simulink library "DEM_lib"  (Simulink 7.4)
settings: Solver=FixedStepDiscrete  StartTime=0.0  StopTime=Inf  FixedStep=0.001  RelTol=1e-3
undefined symbols (not defined in the file or in its folder): BCU_Drive_St, BCU_FastCharge_St, BCU_SlowCharge_St, COR_Fault_Bus, CTC_DefaultOffline_CtrCmd, CTC_DriveEmgyDcnct_CtrCmd, CTC_DriveOffline_CtrCmd, CTC_DriveOnline_CtrCmd, EHP_Fault_Bus, FCM_Fault_Bus, SCM_Fault_Bus
libraries: Defined_Functionality x82, simulink x2
(part 2 of 4)

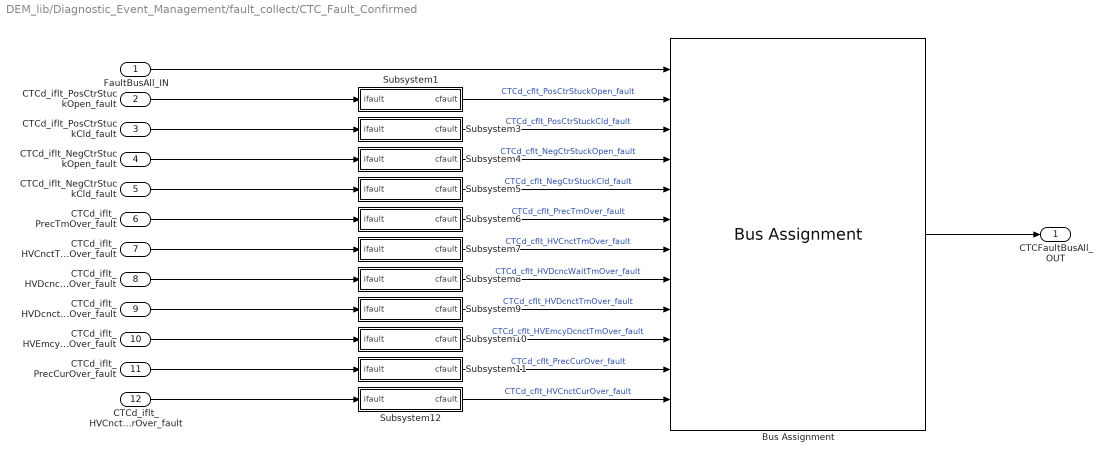
== system DEM_lib/Diagnostic_Event_Management/fault_collect/CTC_Fault_Confirmed ==
  FaultBusAll_IN : Inport
  CTCd_iflt_PosCtrStuckOpen_fault : Inport  Port=2
  CTCd_iflt_PosCtrStuckCld_fault : Inport  Port=3
  CTCd_iflt_NegCtrStuckOpen_fault : Inport  Port=4
  CTCd_iflt_NegCtrStuckCld_fault : Inport  Port=5
  CTCd_iflt_PrecTmOver_fault : Inport  Port=6
  CTCd_iflt_HVCnctTmOver_fault : Inport  Port=7
  CTCd_iflt_HVDcncWaitTmOver_fault : Inport  Port=8
  CTCd_iflt_HVDcnctTmOver_fault : Inport  Port=9
  CTCd_iflt_HVEmcyDcnctTmOver_fault : Inport  Port=10
  CTCd_iflt_PrecCurOver_fault : Inport  Port=11
  CTCd_iflt_HVCnctCurOver_fault : Inport  Port=12
  Bus Assignment : BusAssignment  Description=|  AssignedSignals=CTC_Fault_Bus.CTCd_cflt_PosCtrStuckOpen_faultRaw,CTC_Fault_Bus.CTCd_cflt_PosCtrStuckCld_faultRaw,CTC_Fault_Bus.CTCd_cflt_NegCtrStuckOpen_faultRaw,CTC_Fault_Bus.CTCd_cflt_NegCtrStuckCld_faultRaw,CTC_Fault_Bus.CTCd_cflt_PrecTmOver_faultRaw,CTC_Fault_Bus.CTCd_cflt_HVCnctTmOver_faultRaw,CTC_Fault_Bus.CTCd_cflt_HVDcncWaitTmOver_faultRaw,CTC_Fault_Bus.CTCd_cflt_HVDcnctTmOver_faultRaw,CTC_Fault_Bus.CTCd_cflt_HVEmcyDcnctTmOver_faultRaw,CTC_Fault_Bus.CTCd_cflt_PrecCurOver_faultRaw,CTC_Fault_Bus.CTCd_cflt_HVCnctCurOver_faultRaw
      | $Author:Yan LiJuan$
      | $Date:2015/03/26$  
      | $Revision:1.0$
  Subsystem1 : Subsystem
  Subsystem10 : Subsystem
  Subsystem11 : Subsystem
  Subsystem12 : Subsystem
  Subsystem3 : Subsystem
  Subsystem4 : Subsystem
  Subsystem5 : Subsystem
  Subsystem6 : Subsystem
  Subsystem7 : Subsystem
  Subsystem8 : Subsystem
  Subsystem9 : Subsystem
  CTCFaultBusAll_OUT : Outport
  wires:
  Subsystem12/1(cfault) -> Bus Assignment/12  "CTCd_cflt_HVCnctCurOver_fault"
  Subsystem11/1(cfault) -> Bus Assignment/11  "CTCd_cflt_PrecCurOver_fault"
  Subsystem10/1(cfault) -> Bus Assignment/10  "CTCd_cflt_HVEmcyDcnctTmOver_fault"
  Subsystem9/1(cfault) -> Bus Assignment/9  "CTCd_cflt_HVDcnctTmOver_fault"
  Subsystem8/1(cfault) -> Bus Assignment/8  "CTCd_cflt_HVDcncWaitTmOver_fault"
  Subsystem7/1(cfault) -> Bus Assignment/7  "CTCd_cflt_HVCnctTmOver_fault"
  Subsystem6/1(cfault) -> Bus Assignment/6  "CTCd_cflt_PrecTmOver_fault"
  Subsystem5/1(cfault) -> Bus Assignment/5  "CTCd_cflt_NegCtrStuckCld_fault"
  Subsystem4/1(cfault) -> Bus Assignment/4  "CTCd_cflt_NegCtrStuckOpen_fault"
  Subsystem3/1(cfault) -> Bus Assignment/3  "CTCd_cflt_PosCtrStuckCld_fault"
  Subsystem1/1(cfault) -> Bus Assignment/2  "CTCd_cflt_PosCtrStuckOpen_fault"
  Bus Assignment/1 -> CTCFaultBusAll_OUT/1
  CTCd_iflt_HVCnctCurOver_fault/1 -> Subsystem12/1(ifault)
  CTCd_iflt_PrecCurOver_fault/1 -> Subsystem11/1(ifault)
  CTCd_iflt_HVEmcyDcnctTmOver_fault/1 -> Subsystem10/1(ifault)
  CTCd_iflt_HVDcnctTmOver_fault/1 -> Subsystem9/1(ifault)
  CTCd_iflt_HVDcncWaitTmOver_fault/1 -> Subsystem8/1(ifault)
  CTCd_iflt_HVCnctTmOver_fault/1 -> Subsystem7/1(ifault)
  CTCd_iflt_PrecTmOver_fault/1 -> Subsystem6/1(ifault)
  CTCd_iflt_NegCtrStuckCld_fault/1 -> Subsystem5/1(ifault)
  CTCd_iflt_NegCtrStuckOpen_fault/1 -> Subsystem4/1(ifault)
  CTCd_iflt_PosCtrStuckCld_fault/1 -> Subsystem3/1(ifault)
  CTCd_iflt_PosCtrStuckOpen_fault/1 -> Subsystem1/1(ifault)
  FaultBusAll_IN/1 -> Bus Assignment/1

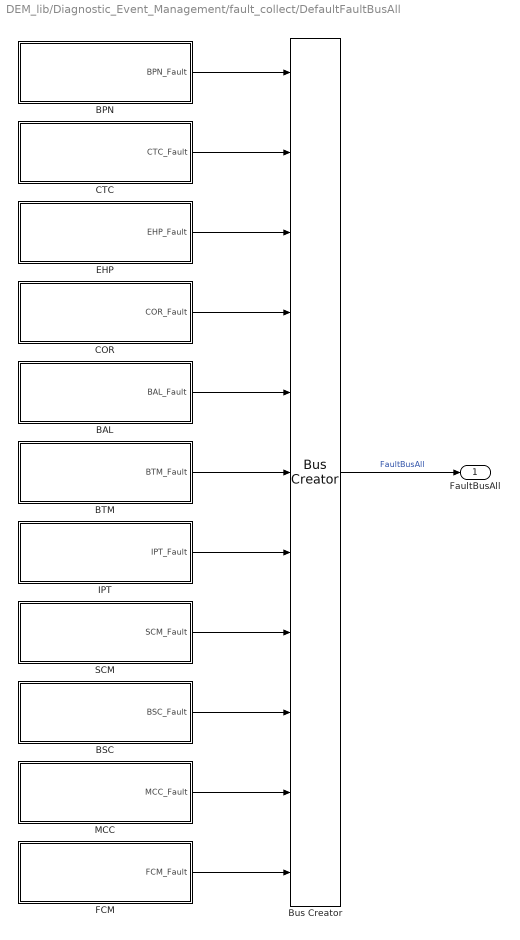
== system DEM_lib/Diagnostic_Event_Management/fault_collect/DefaultFaultBusAll ==
  BAL : Subsystem  Description=|
      | $Author:Yan LiJuan$
      | $Date:2015/03/26$  
      | $Revision:1.0$
  BPN : Subsystem  Description=|
      | $Author:Yan LiJuan$
      | $Date:2015/03/26$  
      | $Revision:1.0$
  BSC : Subsystem  Description=|
      | $Author:Yan LiJuan$
      | $Date:2015/03/26$  
      | $Revision:1.0$
  BTM : Subsystem  Description=|
      | $Author:Yan LiJuan$
      | $Date:2015/03/26$  
      | $Revision:1.0$
  Bus Creator : BusCreator  Inputs=11
  COR : Subsystem  Description=|
      | $Author:Yan LiJuan$
      | $Date:2015/03/26$  
      | $Revision:1.0$
  CTC : Subsystem  Description=|
      | $Author:Yan LiJuan$
      | $Date:2015/03/26$  
      | $Revision:1.0$
  EHP : Subsystem  Description=|
      | $Author:Yan LiJuan$
      | $Date:2015/03/26$  
      | $Revision:1.0$
  FCM : Subsystem  Description=|
      | $Author:Yan LiJuan$
      | $Date:2015/03/26$  
      | $Revision:1.0$
  IPT : Subsystem  Description=|
      | $Author:Yan LiJuan$
      | $Date:2015/03/26$  
      | $Revision:1.0$
  MCC : Subsystem  Description=|
      | $Author:Yan LiJuan$
      | $Date:2015/03/26$  
      | $Revision:1.0$
  SCM : Subsystem  Description=|
      | $Author:Yan LiJuan$
      | $Date:2015/03/26$  
      | $Revision:1.0$
  FaultBusAll : Outport  OutDataType=fixdt(1, 16)  OutScaling=2^0
  wires:
  FCM/1(FCM_Fault) -> Bus Creator/11
  BSC/1(BSC_Fault) -> Bus Creator/9
  SCM/1(SCM_Fault) -> Bus Creator/8
  Bus Creator/1 -> FaultBusAll/1  "FaultBusAll"
  IPT/1(IPT_Fault) -> Bus Creator/7
  BTM/1(BTM_Fault) -> Bus Creator/6
  BAL/1(BAL_Fault) -> Bus Creator/5
  COR/1(COR_Fault) -> Bus Creator/4
  EHP/1(EHP_Fault) -> Bus Creator/3
  CTC/1(CTC_Fault) -> Bus Creator/2
  BPN/1(BPN_Fault) -> Bus Creator/1
  MCC/1(MCC_Fault) -> Bus Creator/10

== system DEM_lib/Diagnostic_Event_Management/fault_collect/EHP_Fault_Confirmed ==
  FaultBusAll_IN : Inport
  EHPd_iflt_NegIso_fault : Inport  Port=2
  EHPd_iflt_NegIso_warn : Inport  Port=3
  EHPd_iflt_PosIso_fault : Inport  Port=4
  EHPd_iflt_PosIso_warn : Inport  Port=5
  EHPd_iflt_HVILSt_fault : Inport  Port=6
  Bus Assignment : BusAssignment  Description=|  AssignedSignals=EHP_Fault_Bus.EHPd_cflt_NegIso_faultRaw,EHP_Fault_Bus.EHPd_cflt_NegIso_warnRaw,EHP_Fault_Bus.EHPd_cflt_PosIso_faultRaw,EHP_Fault_Bus.EHPd_cflt_PosIso_warnRaw,EHP_Fault_Bus.EHPd_cflt_HVILSt_faultRaw
      | $Author:Yan LiJuan$
      | $Date:2015/03/26$  
      | $Revision:1.0$
  Subsystem2 : Subsystem
  Subsystem4 : Subsystem
  Subsystem5 : Subsystem
  Subsystem6 : Subsystem
  Subsystem7 : Subsystem
  EHPFaultBusAll_OUT : Outport
  wires:
  Subsystem7/1(cfault) -> Bus Assignment/6  "EHPd_cflt_HVILSt_fault"
  Subsystem6/1(cfault) -> Bus Assignment/5  "EHPd_cflt_PosIso_warn"
  Subsystem5/1(cfault) -> Bus Assignment/4  "EHPd_cflt_PosIso_fault"
  Subsystem4/1(cfault) -> Bus Assignment/3  "EHPd_cflt_NegIso_warn"
  Subsystem2/1(cfault) -> Bus Assignment/2  "EHPd_cflt_NegIso_fault"
  EHPd_iflt_HVILSt_fault/1 -> Subsystem7/1(ifault)
  EHPd_iflt_PosIso_warn/1 -> Subsystem6/1(ifault)
  EHPd_iflt_PosIso_fault/1 -> Subsystem5/1(ifault)
  EHPd_iflt_NegIso_warn/1 -> Subsystem4/1(ifault)
  EHPd_iflt_NegIso_fault/1 -> Subsystem2/1(ifault)
  Bus Assignment/1 -> EHPFaultBusAll_OUT/1
  FaultBusAll_IN/1 -> Bus Assignment/1

== system DEM_lib/Diagnostic_Event_Management/fault_collect/FCM_Fault_Confirmed ==
  FaultBusAll_IN : Inport
  FCMd_iflt_ChaCurDifOver_fault : Inport  Port=2
  FCMd_iflt_ChaVoltDifOver_fault : Inport  Port=3
  Bus Assignment : BusAssignment  Description=|  AssignedSignals=FCM_Fault_Bus.FCMd_cflt_ChaCurDifOver_faultRaw,FCM_Fault_Bus.FCMd_cflt_ChaVoltDifOver_faultRaw
      | $Author:Yan LiJuan$
      | $Date:2015/03/26$  
      | $Revision:1.0$
  Subsystem1 : Subsystem
  Subsystem2 : Subsystem
  FCMIPTFaultBusAll_OUT : Outport
  wires:
  Subsystem2/1(cfault) -> Bus Assignment/2  "FCMd_cflt_ChaCurDifOver_fault"
  Subsystem1/1(cfault) -> Bus Assignment/3  "FCMd_cflt_ChaVoltDifOver_fault"
  FCMd_iflt_ChaVoltDifOver_fault/1 -> Subsystem1/1(ifault)
  FCMd_iflt_ChaCurDifOver_fault/1 -> Subsystem2/1(ifault)
  Bus Assignment/1 -> FCMIPTFaultBusAll_OUT/1  "FCMIPTFaultBusAll_OUT"
  FaultBusAll_IN/1 -> Bus Assignment/1

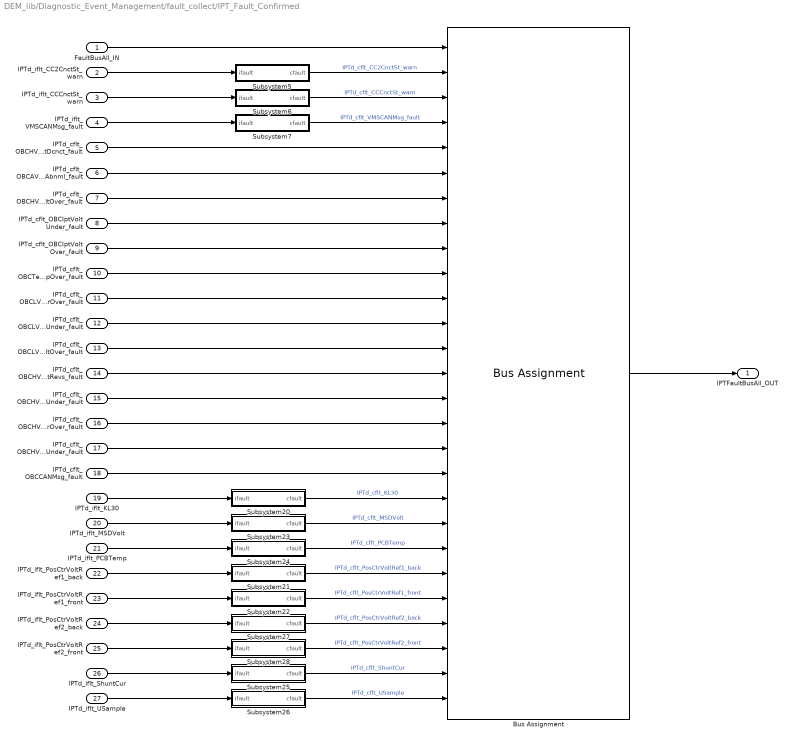
== system DEM_lib/Diagnostic_Event_Management/fault_collect/IPT_Fault_Confirmed ==
  FaultBusAll_IN : Inport
  IPTd_iflt_CC2CnctSt_warn : Inport  Port=2
  IPTd_iflt_CCCnctSt_warn : Inport  Port=3
  IPTd_iflt_VMSCANMsg_fault : Inport  Port=4
  IPTd_cflt_OBCHVOptDcnct_fault : Inport  Port=5  OutDataType=fixdt(1, 16)  OutScaling=2^0
  IPTd_cflt_OBCAVOptVoltAbnml_fault : Inport  Port=6  OutDataType=fixdt(1, 16)  OutScaling=2^0
  IPTd_cflt_OBCHVOptVoltOver_fault : Inport  Port=7  OutDataType=fixdt(1, 16)  OutScaling=2^0
  IPTd_cflt_OBCIptVoltUnder_fault : Inport  Port=8  OutDataType=fixdt(1, 16)  OutScaling=2^0
  IPTd_cflt_OBCIptVoltOver_fault : Inport  Port=9  OutDataType=fixdt(1, 16)  OutScaling=2^0
  IPTd_cflt_OBCTempOver_fault : Inport  Port=10  OutDataType=fixdt(1, 16)  OutScaling=2^0
  IPTd_cflt_OBCLVOptCurOver_fault : Inport  Port=11  OutDataType=fixdt(1, 16)  OutScaling=2^0
  IPTd_cflt_OBCLVOptVoltUnder_fault : Inport  Port=12  OutDataType=fixdt(1, 16)  OutScaling=2^0
  IPTd_cflt_OBCLVOptVoltOver_fault : Inport  Port=13  OutDataType=fixdt(1, 16)  OutScaling=2^0
  IPTd_cflt_OBCHVOptRevs_fault : Inport  Port=14  OutDataType=fixdt(1, 16)  OutScaling=2^0
  IPTd_cflt_OBCHVOptCurUnder_fault : Inport  Port=15  OutDataType=fixdt(1, 16)  OutScaling=2^0
  IPTd_cflt_OBCHVOptCurOver_fault : Inport  Port=16  OutDataType=fixdt(1, 16)  OutScaling=2^0
  IPTd_cflt_OBCHVOptVoltUnder_fault : Inport  Port=17  OutDataType=fixdt(1, 16)  OutScaling=2^0
  IPTd_cflt_OBCCANMsg_fault : Inport  Port=18  OutDataType=fixdt(1, 16)  OutScaling=2^0
  IPTd_iflt_KL30 : Inport  Port=19  OutDataType=fixdt(1, 16)  OutScaling=2^0
  IPTd_iflt_MSDVolt : Inport  Port=20  OutDataType=fixdt(1, 16)  OutScaling=2^0
  IPTd_iflt_PCBTemp : Inport  Port=21  OutDataType=fixdt(1, 16)  OutScaling=2^0
  IPTd_iflt_PosCtrVoltRef1_back : Inport  Port=22  OutDataType=fixdt(1, 16)  OutScaling=2^0
  IPTd_iflt_PosCtrVoltRef1_front : Inport  Port=23  OutDataType=fixdt(1, 16)  OutScaling=2^0
  IPTd_iflt_PosCtrVoltRef2_back : Inport  Port=24  OutDataType=fixdt(1, 16)  OutScaling=2^0
  IPTd_iflt_PosCtrVoltRef2_front : Inport  Port=25  OutDataType=fixdt(1, 16)  OutScaling=2^0
  IPTd_iflt_ShuntCur : Inport  Port=26  OutDataType=fixdt(1, 16)  OutScaling=2^0
  IPTd_iflt_USample : Inport  Port=27  OutDataType=fixdt(1, 16)  OutScaling=2^0
  Bus Assignment : BusAssignment  Description=|  AssignedSignals=IPT_Fault_Bus.IPTd_cflt_CC2CnctSt_warnRaw,IPT_Fault_Bus.IPTd_cflt_CCCnctSt_warnRaw,IPT_Fault_Bus.IPTd_cflt_VMSCANMsg_faultRaw,IPT_Fault_Bus.IPTd_cflt_OBCHVOptDcnct_faultRaw,IPT_Fault_Bus.IPTd_cflt_OBCAVOptVoltAbnml_faultRaw,IPT_Fault_Bus.IPTd_cflt_OBCHVOptVoltOver_faultRaw,IPT_Fault_Bus.IPTd_cflt_OBCIptVoltUnder_faultRaw,IPT_Fault_Bus.IPTd_cflt_OBCIptVoltOver_faultRaw,IPT_Fault_Bus.IPTd_cflt_OBCTempOver_faultRaw,IPT_Fault_Bus.IPTd_cflt_OBCLVOptCurOver_faultRaw,IPT_Fault_Bus.IPTd_cflt_OBCLVOptVoltUnder_faultRaw,IPT_Fault_Bus.IPTd_cflt_OBCLVOptVoltOver_faultRaw,IPT_Fault_Bus.IPTd_cflt_OBCHVOptRevs_faultRaw,IPT_Fault_Bus.IPTd_cflt_OBCHVOptCurUnder_faultRaw,IPT_Fault_Bus.IPTd_cflt_OBCHVOptCurOver_faultRaw,IPT_Fault_Bus.IPTd_cflt_OBCHVOptVoltUnder_faultRaw,IPT_Fault_Bus.IPTd_cflt_OBCCANMsg_faultRaw,IPT_Fault_Bus.IPTd_cflt_KL30Raw,IPT_Fault_Bus.IPTd_cflt_MSDVoltRaw,IPT_Fault_Bus.IPTd_cflt_PCBTempRaw,IPT_Fault_Bus.IPTd_cflt_PosCtrVoltRef1_backRaw,IPT_Fault_Bus.IPTd_cflt_PosCtrVoltRef1_frontRaw,IPT_Fault_Bus.IPTd_cflt_PosCtrVoltRef2_backRaw,IPT_Fault_Bus.IPTd_cflt_PosCtrVoltRef2_frontRaw,IPT_Fault_Bus.IPTd_cflt_ShuntCurRaw,IPT_Fault_Bus.IPTd_cflt_USampleRaw
      | $Author:Yan LiJuan$
      | $Date:2015/03/26$  
      | $Revision:1.0$
  Subsystem20 : Subsystem
  Subsystem21 : Subsystem
  Subsystem22 : Subsystem
  Subsystem23 : Subsystem
  Subsystem24 : Subsystem
  Subsystem25 : Subsystem
  Subsystem26 : Subsystem
  Subsystem27 : Subsystem
  Subsystem28 : Subsystem
  Subsystem5 : Subsystem
  Subsystem6 : Subsystem
  Subsystem7 : Subsystem
  IPTFaultBusAll_OUT : Outport
  wires:
  IPTd_cflt_OBCAVOptVoltAbnml_fault/1 -> Bus Assignment/6
  IPTd_cflt_OBCHVOptDcnct_fault/1 -> Bus Assignment/5
  Subsystem7/1(cfault) -> Bus Assignment/4  "IPTd_cflt_VMSCANMsg_fault"
  Subsystem6/1(cfault) -> Bus Assignment/3  "IPTd_cflt_CCCnctSt_warn"
  Subsystem5/1(cfault) -> Bus Assignment/2  "IPTd_cflt_CC2CnctSt_warn"
  IPTd_iflt_VMSCANMsg_fault/1 -> Subsystem7/1(ifault)
  IPTd_iflt_CCCnctSt_warn/1 -> Subsystem6/1(ifault)
  IPTd_iflt_CC2CnctSt_warn/1 -> Subsystem5/1(ifault)
  Bus Assignment/1 -> IPTFaultBusAll_OUT/1
  FaultBusAll_IN/1 -> Bus Assignment/1
  Subsystem20/1(cfault) -> Bus Assignment/19  "IPTd_cflt_KL30"
  Subsystem23/1(cfault) -> Bus Assignment/20  "IPTd_cflt_MSDVolt"
  Subsystem24/1(cfault) -> Bus Assignment/21  "IPTd_cflt_PCBTemp"
  Subsystem21/1(cfault) -> Bus Assignment/22  "IPTd_cflt_PosCtrVoltRef1_back"
  Subsystem22/1(cfault) -> Bus Assignment/23  "IPTd_cflt_PosCtrVoltRef1_front"
  Subsystem27/1(cfault) -> Bus Assignment/24  "IPTd_cflt_PosCtrVoltRef2_back"
  Subsystem28/1(cfault) -> Bus Assignment/25  "IPTd_cflt_PosCtrVoltRef2_front"
  Subsystem25/1(cfault) -> Bus Assignment/26  "IPTd_cflt_ShuntCur"
  Subsystem26/1(cfault) -> Bus Assignment/27  "IPTd_cflt_USample"
  IPTd_iflt_KL30/1 -> Subsystem20/1(ifault)
  IPTd_iflt_MSDVolt/1 -> Subsystem23/1(ifault)
  IPTd_iflt_PCBTemp/1 -> Subsystem24/1(ifault)
  IPTd_iflt_PosCtrVoltRef1_back/1 -> Subsystem21/1(ifault)
  IPTd_iflt_PosCtrVoltRef1_front/1 -> Subsystem22/1(ifault)
  IPTd_iflt_PosCtrVoltRef2_back/1 -> Subsystem27/1(ifault)
  IPTd_iflt_PosCtrVoltRef2_front/1 -> Subsystem28/1(ifault)
  IPTd_iflt_ShuntCur/1 -> Subsystem25/1(ifault)
  IPTd_iflt_USample/1 -> Subsystem26/1(ifault)
  IPTd_cflt_OBCHVOptVoltOver_fault/1 -> Bus Assignment/7
  IPTd_cflt_OBCIptVoltUnder_fault/1 -> Bus Assignment/8
  IPTd_cflt_OBCIptVoltOver_fault/1 -> Bus Assignment/9
  IPTd_cflt_OBCTempOver_fault/1 -> Bus Assignment/10
  IPTd_cflt_OBCLVOptCurOver_fault/1 -> Bus Assignment/11
  IPTd_cflt_OBCLVOptVoltUnder_fault/1 -> Bus Assignment/12
  IPTd_cflt_OBCLVOptVoltOver_fault/1 -> Bus Assignment/13
  IPTd_cflt_OBCHVOptRevs_fault/1 -> Bus Assignment/14
  IPTd_cflt_OBCHVOptCurUnder_fault/1 -> Bus Assignment/15
  IPTd_cflt_OBCHVOptCurOver_fault/1 -> Bus Assignment/16
  IPTd_cflt_OBCHVOptVoltUnder_fault/1 -> Bus Assignment/17
  IPTd_cflt_OBCCANMsg_fault/1 -> Bus Assignment/18

== system DEM_lib/Diagnostic_Event_Management/fault_collect/MCC_Fault_Confirmed ==
  FaultBusAll_IN : Inport
  MCCd_iflt_BMUInit_fault : Inport  Port=2
  Bus Assignment : BusAssignment  Description=|  AssignedSignals=MCC_Fault_Bus.MCCd_cflt_BMUInit_faultRaw
      | $Author:Yan LiJuan$
      | $Date:2015/03/26$  
      | $Revision:1.0$
  Subsystem2 : Subsystem
  MCCFaultBusAll_OUT : Outport
  wires:
  FaultBusAll_IN/1 -> Bus Assignment/1
  Bus Assignment/1 -> MCCFaultBusAll_OUT/1  "MCCFaultBusAll_OUT"
  MCCd_iflt_BMUInit_fault/1 -> Subsystem2/1(ifault)
  Subsystem2/1(cfault) -> Bus Assignment/2  "MCCd_cflt_BMUInit_fault"

== system DEM_lib/Diagnostic_Event_Management/fault_collect/SCM_Fault_Confirmed ==
  FaultBusAll_IN : Inport
  SCMd_iflt_CurOver_fault : Inport  Port=2
  SCMd_iflt_VoltOver_fault : Inport  Port=3
  Bus Assignment : BusAssignment  Description=|  AssignedSignals=SCM_Fault_Bus.SCMd_cflt_CurOver_faultRaw,SCM_Fault_Bus.SCMd_cflt_VoltOver_faultRaw
      | $Author:Yan LiJuan$
      | $Date:2015/03/26$  
      | $Revision:1.0$
  Subsystem1 : Subsystem
  Subsystem2 : Subsystem
  SCMFaultBusAll_OUT : Outport
  wires:
  FaultBusAll_IN/1 -> Bus Assignment/1
  Bus Assignment/1 -> SCMFaultBusAll_OUT/1  "SCMFaultBusAll_OUT"
  SCMd_iflt_CurOver_fault/1 -> Subsystem2/1(ifault)
  SCMd_iflt_VoltOver_fault/1 -> Subsystem1/1(ifault)
  Subsystem2/1(cfault) -> Bus Assignment/2  "SCMd_cflt_CurOver_fault"
  Subsystem1/1(cfault) -> Bus Assignment/3  "SCMd_cflt_VoltOver_fault"

== system DEM_lib/Diagnostic_Event_Management/Level_handle/DRIVE/FaultLevelConfirmed ==
  DEMd_cflt_fault : Inport
  LvlErr1 : Subsystem
  LvlErr2 : Subsystem
  LvlErr3 : Subsystem
  MinMax : MinMax  Function=max  Inputs=3
  signal_debug : Defined_Functionality/signal_debug  SystemSampleTime=-1  debug_switch=DEMc_dbgsw_FaultLev  debug_value=DEMc_dbgval_FaultLev
      settings: AttributesFormatString=[SWITCH=%<debug_switch>]\n[VALUE=%<debug_value>]
  DEMd_enum_FaultLev : Outport
  wires:
  signal_debug/1 -> DEMd_enum_FaultLev/1  "DEMd_enum_FaultLev"
  MinMax/1 -> signal_debug/1  "DEMd_enum_FaultLevRaw"
  LvlErr3/1(ErrLvl) -> MinMax/3
  LvlErr2/1(ErrLvl) -> MinMax/2
  LvlErr1/1(ErrLvl) -> MinMax/1
  DEMd_cflt_fault/1 -> LvlErr3/1(Err), LvlErr2/1(Err), LvlErr1/1(Err)

== system DEM_lib/Diagnostic_Event_Management/Level_handle/DRIVE/handle ==
  DEMd_enum_FaultLev : Inport
  DEMd_cflt_fault : Inport  Port=2
  IPTd_flg_VehHVCnctCmd : Inport  Port=3
  BSCd_enum_BCUSt : Inport  Port=4
  DriveCtrCmdRaw : Subsystem  Description=|
      | $Author:Yan LiJuan$
      | $Date:2015/03/26$  
      | $Revision:1.0$
  Subsystem : Subsystem  Description=|
      | $Author:Yan LiJuan$
      | $Date:2015/09/15$  
      | $Revision:1.1$
  serious 1 : Subsystem  Description=|
      | $Author:Yan LiJuan$
      | $Date:2015/09/15$  
      | $Revision:1.1$
  DEMd_enum_CtrCmdRaw : Outport
  DEMd_flg_HVdcnctReq : Outport  Port=2
  DEMd_flg_TmOverWarn : Outport  Port=3
  wires:
  IPTd_flg_VehHVCnctCmd/1 -> Subsystem/3(IPTd_flg_VehHVCnctCmd), DriveCtrCmdRaw/2(IPTd_flg_VehHVCnctCmd)
  Subsystem/2(DEMd_flg_HVdcnctReq) -> DEMd_flg_HVdcnctReq/1
  Subsystem/3(DEMd_flg_TmOverWarn) -> DEMd_flg_TmOverWarn/1
  serious 1/1(DEMd_enum_CtrCmdRaw) -> DEMd_enum_CtrCmdRaw/1
  Subsystem/1(DEMd_enum_DrvCtrCmd) -> serious 1/3(DEMd_enum_DrvCtrCmd)
  DriveCtrCmdRaw/1(DEMd_enum_DrvCtrCmdRaw) -> Subsystem/2(DEMd_enum_DrvCtrCmdRaw)
  DEMd_enum_FaultLev/1 -> serious 1/2(DEMd_enum_FaultLev), Subsystem/1(DEMd_enum_FaultLev)
  DEMd_cflt_fault/1 -> serious 1/1(DEMd_cflt_fault)
  BSCd_enum_BCUSt/1 -> DriveCtrCmdRaw/1(BSCd_enum_BCUSt)

== system DEM_lib/Diagnostic_Event_Management/fault_collect/BAL_Fault_Confirmed/Subsystem2 ==
  ifault : Inport  OutDataType=fixdt(1, 16)  OutScaling=2^0
  Terminator : Terminator
  Terminator1 : Terminator
  Terminator2 : Terminator
  diagnostic1 : Defined_Functionality/diagnostic1  SystemSampleTime=-1  afl_inc=DEMc_BalSwthAnmlwarn_inc  afl_dec=DEMc_BalSwthAnmlwarn_dec  afl_threshold=DEMc_BalSwthAnmlwarn_AflThrld  aff_threshold=DEMc_BalSwthAnmlwarn_AffThrld
      settings: AttributesFormatString=[AFL_INCREMENT=%<afl_inc>]\n[AFL_DECREMENT=%<afl_dec>]\n[AFL_THRESHOLD=%<afl_threshold>]\n[AFF_THRESHOLD=%<aff_threshold>]
  cfault : Outport  OutDataType=fixdt(1, 16)  OutScaling=2^0
  wires:
  diagnostic1/3 -> Terminator2/1
  diagnostic1/4 -> Terminator1/1
  diagnostic1/1 -> Terminator/1
  diagnostic1/2 -> cfault/1
  ifault/1 -> diagnostic1/1

== system DEM_lib/Diagnostic_Event_Management/fault_collect/BPN_Fault_Confirmed/CellVoltOver_warn ==
  ifault : Inport  OutDataType=fixdt(1, 16)  OutScaling=2^0
  Terminator : Terminator
  Terminator1 : Terminator
  Terminator2 : Terminator
  diagnostic1 : Defined_Functionality/diagnostic1  Description=|  SystemSampleTime=-1  afl_inc=DEMc_CellVoltOverwarn_inc  afl_dec=DEMc_CellVoltOverwarn_dec  afl_threshold=DEMc_CellVoltOverwarn_AflThrld  aff_threshold=DEMc_CellVoltOverwarn_AffThrld
      | $Author:Yan LiJuan$
      | $Date:2015/03/26$  
      | $Revision:1.0$
      settings: AttributesFormatString=[AFL_INCREMENT=%<afl_inc>]\n[AFL_DECREMENT=%<afl_dec>]\n[AFL_THRESHOLD=%<afl_threshold>]\n[AFF_THRESHOLD=%<aff_threshold>]
  cfault : Outport  OutDataType=fixdt(1, 16)  OutScaling=2^0
  wires:
  ifault/1 -> diagnostic1/1
  diagnostic1/2 -> cfault/1
  diagnostic1/1 -> Terminator/1
  diagnostic1/4 -> Terminator1/1
  diagnostic1/3 -> Terminator2/1

== system DEM_lib/Diagnostic_Event_Management/fault_collect/BPN_Fault_Confirmed/Subsystem11 ==
  ifault : Inport  OutDataType=fixdt(1, 16)  OutScaling=2^0
  Terminator : Terminator
  Terminator1 : Terminator
  Terminator2 : Terminator
  diagnostic1 : Defined_Functionality/diagnostic1  SystemSampleTime=-1  afl_inc=DEMc_PackVoltOverwarn_inc  afl_dec=DEMc_PackVoltOverwarn_dec  afl_threshold=DEMc_PackVoltOverwarn_AflThrld  aff_threshold=DEMc_PackVoltOverwarn_AffThrld
      settings: AttributesFormatString=[AFL_INCREMENT=%<afl_inc>]\n[AFL_DECREMENT=%<afl_dec>]\n[AFL_THRESHOLD=%<afl_threshold>]\n[AFF_THRESHOLD=%<aff_threshold>]
  cfault : Outport  OutDataType=fixdt(1, 16)  OutScaling=2^0
  wires:
  diagnostic1/3 -> Terminator2/1
  diagnostic1/4 -> Terminator1/1
  diagnostic1/1 -> Terminator/1
  diagnostic1/2 -> cfault/1
  ifault/1 -> diagnostic1/1

== system DEM_lib/Diagnostic_Event_Management/fault_collect/BPN_Fault_Confirmed/Subsystem12 ==
  ifault : Inport  OutDataType=fixdt(1, 16)  OutScaling=2^0
  Terminator : Terminator
  Terminator1 : Terminator
  Terminator2 : Terminator
  diagnostic1 : Defined_Functionality/diagnostic1  SystemSampleTime=-1  afl_inc=DEMc_PackVoltOverfault_inc  afl_dec=DEMc_PackVoltOverfault_dec  afl_threshold=DEMc_PackVoltOverfault_AflThrld  aff_threshold=DEMc_PackVoltOverfault_AffThrld
      settings: AttributesFormatString=[AFL_INCREMENT=%<afl_inc>]\n[AFL_DECREMENT=%<afl_dec>]\n[AFL_THRESHOLD=%<afl_threshold>]\n[AFF_THRESHOLD=%<aff_threshold>]
  cfault : Outport  OutDataType=fixdt(1, 16)  OutScaling=2^0
  wires:
  ifault/1 -> diagnostic1/1
  diagnostic1/2 -> cfault/1
  diagnostic1/1 -> Terminator/1
  diagnostic1/4 -> Terminator1/1
  diagnostic1/3 -> Terminator2/1

== system DEM_lib/Diagnostic_Event_Management/fault_collect/BPN_Fault_Confirmed/Subsystem13 ==
  ifault : Inport  OutDataType=fixdt(1, 16)  OutScaling=2^0
  Terminator : Terminator
  Terminator1 : Terminator
  Terminator2 : Terminator
  diagnostic1 : Defined_Functionality/diagnostic1  SystemSampleTime=-1  afl_inc=DEMc_PackVoltOverfatal_inc  afl_dec=DEMc_PackVoltOverfatal_dec  afl_threshold=DEMc_PackVoltOverfatal_AflThrld  aff_threshold=DEMc_PackVoltOverfatal_AffThrld
      settings: AttributesFormatString=[AFL_INCREMENT=%<afl_inc>]\n[AFL_DECREMENT=%<afl_dec>]\n[AFL_THRESHOLD=%<afl_threshold>]\n[AFF_THRESHOLD=%<aff_threshold>]
  cfault : Outport  OutDataType=fixdt(1, 16)  OutScaling=2^0
  wires:
  diagnostic1/3 -> Terminator2/1
  diagnostic1/4 -> Terminator1/1
  diagnostic1/1 -> Terminator/1
  diagnostic1/2 -> cfault/1
  ifault/1 -> diagnostic1/1

== system DEM_lib/Diagnostic_Event_Management/fault_collect/BPN_Fault_Confirmed/Subsystem14 ==
  ifault : Inport  OutDataType=fixdt(1, 16)  OutScaling=2^0
  Terminator : Terminator
  Terminator1 : Terminator
  Terminator2 : Terminator
  diagnostic1 : Defined_Functionality/diagnostic1  SystemSampleTime=-1  afl_inc=DEMc_PackVoltUnderwarn_inc  afl_dec=DEMc_PackVoltUnderwarn_dec  afl_threshold=DEMc_PackVoltUnderwarn_AflThrld  aff_threshold=DEMc_PackVoltUnderwarn_AffThrld
      settings: AttributesFormatString=[AFL_INCREMENT=%<afl_inc>]\n[AFL_DECREMENT=%<afl_dec>]\n[AFL_THRESHOLD=%<afl_threshold>]\n[AFF_THRESHOLD=%<aff_threshold>]
  cfault : Outport  OutDataType=fixdt(1, 16)  OutScaling=2^0
  wires:
  ifault/1 -> diagnostic1/1
  diagnostic1/2 -> cfault/1
  diagnostic1/1 -> Terminator/1
  diagnostic1/4 -> Terminator1/1
  diagnostic1/3 -> Terminator2/1

== system DEM_lib/Diagnostic_Event_Management/fault_collect/BPN_Fault_Confirmed/Subsystem15 ==
  ifault : Inport  OutDataType=fixdt(1, 16)  OutScaling=2^0
  Terminator : Terminator
  Terminator1 : Terminator
  Terminator2 : Terminator
  diagnostic1 : Defined_Functionality/diagnostic1  SystemSampleTime=-1  afl_inc=DEMc_PackVoltUnderfault_inc  afl_dec=DEMc_PackVoltUnderfault_dec  afl_threshold=DEMc_PackVoltUnderfault_AflThrld  aff_threshold=DEMc_PackVoltUnderfault_AffThrld
      settings: AttributesFormatString=[AFL_INCREMENT=%<afl_inc>]\n[AFL_DECREMENT=%<afl_dec>]\n[AFL_THRESHOLD=%<afl_threshold>]\n[AFF_THRESHOLD=%<aff_threshold>]
  cfault : Outport  OutDataType=fixdt(1, 16)  OutScaling=2^0
  wires:
  diagnostic1/3 -> Terminator2/1
  diagnostic1/4 -> Terminator1/1
  diagnostic1/1 -> Terminator/1
  diagnostic1/2 -> cfault/1
  ifault/1 -> diagnostic1/1

== system DEM_lib/Diagnostic_Event_Management/fault_collect/BPN_Fault_Confirmed/Subsystem16 ==
  ifault : Inport  OutDataType=fixdt(1, 16)  OutScaling=2^0
  Terminator : Terminator
  Terminator1 : Terminator
  Terminator2 : Terminator
  diagnostic1 : Defined_Functionality/diagnostic1  SystemSampleTime=-1  afl_inc=DEMc_PackVoltUnderfatal_inc  afl_dec=DEMc_PackVoltUnderfatal_dec  afl_threshold=DEMc_PackVoltUnderfatal_AflThrld  aff_threshold=DEMc_PackVoltUnderfatal_AffThrld
      settings: AttributesFormatString=[AFL_INCREMENT=%<afl_inc>]\n[AFL_DECREMENT=%<afl_dec>]\n[AFL_THRESHOLD=%<afl_threshold>]\n[AFF_THRESHOLD=%<aff_threshold>]
  cfault : Outport  OutDataType=fixdt(1, 16)  OutScaling=2^0
  wires:
  ifault/1 -> diagnostic1/1
  diagnostic1/2 -> cfault/1
  diagnostic1/1 -> Terminator/1
  diagnostic1/4 -> Terminator1/1
  diagnostic1/3 -> Terminator2/1

== system DEM_lib/Diagnostic_Event_Management/fault_collect/BPN_Fault_Confirmed/Subsystem17 ==
  ifault : Inport  OutDataType=fixdt(1, 16)  OutScaling=2^0
  Terminator : Terminator
  Terminator1 : Terminator
  Terminator2 : Terminator
  diagnostic1 : Defined_Functionality/diagnostic1  SystemSampleTime=-1  afl_inc=DEMc_ChaCurOverwarn_inc  afl_dec=DEMc_ChaCurOverwarn_dec  afl_threshold=DEMc_ChaCurOverwarn_AflThrld  aff_threshold=DEMc_ChaCurOverwarn_AffThrld
      settings: AttributesFormatString=[AFL_INCREMENT=%<afl_inc>]\n[AFL_DECREMENT=%<afl_dec>]\n[AFL_THRESHOLD=%<afl_threshold>]\n[AFF_THRESHOLD=%<aff_threshold>]
  cfault : Outport  OutDataType=fixdt(1, 16)  OutScaling=2^0
  wires:
  diagnostic1/3 -> Terminator2/1
  diagnostic1/4 -> Terminator1/1
  diagnostic1/1 -> Terminator/1
  diagnostic1/2 -> cfault/1
  ifault/1 -> diagnostic1/1

== system DEM_lib/Diagnostic_Event_Management/fault_collect/BPN_Fault_Confirmed/Subsystem18 ==
  ifault : Inport  OutDataType=fixdt(1, 16)  OutScaling=2^0
  Terminator : Terminator
  Terminator1 : Terminator
  Terminator2 : Terminator
  diagnostic1 : Defined_Functionality/diagnostic1  SystemSampleTime=-1  afl_inc=DEMc_ChaCurOverfault_inc  afl_dec=DEMc_ChaCurOverfault_dec  afl_threshold=DEMc_ChaCurOverfault_AflThrld  aff_threshold=DEMc_ChaCurOverfault_AffThrld
      settings: AttributesFormatString=[AFL_INCREMENT=%<afl_inc>]\n[AFL_DECREMENT=%<afl_dec>]\n[AFL_THRESHOLD=%<afl_threshold>]\n[AFF_THRESHOLD=%<aff_threshold>]
  cfault : Outport  OutDataType=fixdt(1, 16)  OutScaling=2^0
  wires:
  ifault/1 -> diagnostic1/1
  diagnostic1/2 -> cfault/1
  diagnostic1/1 -> Terminator/1
  diagnostic1/4 -> Terminator1/1
  diagnostic1/3 -> Terminator2/1

== system DEM_lib/Diagnostic_Event_Management/fault_collect/BPN_Fault_Confirmed/Subsystem19 ==
  ifault : Inport  OutDataType=fixdt(1, 16)  OutScaling=2^0
  Terminator : Terminator
  Terminator1 : Terminator
  Terminator2 : Terminator
  diagnostic1 : Defined_Functionality/diagnostic1  SystemSampleTime=-1  afl_inc=DEMc_ChaCurOverfatal_inc  afl_dec=DEMc_ChaCurOverfatal_dec  afl_threshold=DEMc_ChaCurOverfatal_AflThrld  aff_threshold=DEMc_ChaCurOverfatal_AffThrld
      settings: AttributesFormatString=[AFL_INCREMENT=%<afl_inc>]\n[AFL_DECREMENT=%<afl_dec>]\n[AFL_THRESHOLD=%<afl_threshold>]\n[AFF_THRESHOLD=%<aff_threshold>]
  cfault : Outport  OutDataType=fixdt(1, 16)  OutScaling=2^0
  wires:
  diagnostic1/3 -> Terminator2/1
  diagnostic1/4 -> Terminator1/1
  diagnostic1/1 -> Terminator/1
  diagnostic1/2 -> cfault/1
  ifault/1 -> diagnostic1/1

== system DEM_lib/Diagnostic_Event_Management/fault_collect/BPN_Fault_Confirmed/Subsystem20 ==
  ifault : Inport  OutDataType=fixdt(1, 16)  OutScaling=2^0
  Terminator : Terminator
  Terminator1 : Terminator
  Terminator2 : Terminator
  diagnostic1 : Defined_Functionality/diagnostic1  SystemSampleTime=-1  afl_inc=DEMc_DchCurOverwarn_inc  afl_dec=DEMc_DchCurOverwarn_dec  afl_threshold=DEMc_DchCurOverwarn_AflThrld  aff_threshold=DEMc_DchCurOverwarn_AffThrld
      settings: AttributesFormatString=[AFL_INCREMENT=%<afl_inc>]\n[AFL_DECREMENT=%<afl_dec>]\n[AFL_THRESHOLD=%<afl_threshold>]\n[AFF_THRESHOLD=%<aff_threshold>]
  cfault : Outport  OutDataType=fixdt(1, 16)  OutScaling=2^0
  wires:
  ifault/1 -> diagnostic1/1
  diagnostic1/2 -> cfault/1
  diagnostic1/1 -> Terminator/1
  diagnostic1/4 -> Terminator1/1
  diagnostic1/3 -> Terminator2/1

== system DEM_lib/Diagnostic_Event_Management/fault_collect/BPN_Fault_Confirmed/Subsystem21 ==
  ifault : Inport  OutDataType=fixdt(1, 16)  OutScaling=2^0
  Terminator : Terminator
  Terminator1 : Terminator
  Terminator2 : Terminator
  diagnostic1 : Defined_Functionality/diagnostic1  SystemSampleTime=-1  afl_inc=DEMc_DchCurOverfault_inc  afl_dec=DEMc_DchCurOverfault_dec  afl_threshold=DEMc_DchCurOverfault_AflThrld  aff_threshold=DEMc_DchCurOverfault_AffThrld
      settings: AttributesFormatString=[AFL_INCREMENT=%<afl_inc>]\n[AFL_DECREMENT=%<afl_dec>]\n[AFL_THRESHOLD=%<afl_threshold>]\n[AFF_THRESHOLD=%<aff_threshold>]
  cfault : Outport  OutDataType=fixdt(1, 16)  OutScaling=2^0
  wires:
  diagnostic1/3 -> Terminator2/1
  diagnostic1/4 -> Terminator1/1
  diagnostic1/1 -> Terminator/1
  diagnostic1/2 -> cfault/1
  ifault/1 -> diagnostic1/1

== system DEM_lib/Diagnostic_Event_Management/fault_collect/BPN_Fault_Confirmed/Subsystem22 ==
  ifault : Inport  OutDataType=fixdt(1, 16)  OutScaling=2^0
  Terminator : Terminator
  Terminator1 : Terminator
  Terminator2 : Terminator
  diagnostic1 : Defined_Functionality/diagnostic1  SystemSampleTime=-1  afl_inc=DEMc_DchCurOverfatal_inc  afl_dec=DEMc_DchCurOverfatal_dec  afl_threshold=DEMc_DchCurOverfatal_AflThrld  aff_threshold=DEMc_DchCurOverfatal_AffThrld
      settings: AttributesFormatString=[AFL_INCREMENT=%<afl_inc>]\n[AFL_DECREMENT=%<afl_dec>]\n[AFL_THRESHOLD=%<afl_threshold>]\n[AFF_THRESHOLD=%<aff_threshold>]
  cfault : Outport  OutDataType=fixdt(1, 16)  OutScaling=2^0
  wires:
  ifault/1 -> diagnostic1/1
  diagnostic1/2 -> cfault/1
  diagnostic1/1 -> Terminator/1
  diagnostic1/4 -> Terminator1/1
  diagnostic1/3 -> Terminator2/1

== system DEM_lib/Diagnostic_Event_Management/fault_collect/BPN_Fault_Confirmed/Subsystem23 ==
  ifault : Inport  OutDataType=fixdt(1, 16)  OutScaling=2^0
  Terminator : Terminator
  Terminator1 : Terminator
  Terminator2 : Terminator
  diagnostic1 : Defined_Functionality/diagnostic1  SystemSampleTime=-1  afl_inc=DEMc_PackSocUnderwarn_inc  afl_dec=DEMc_PackSocUnderwarn_dec  afl_threshold=DEMc_PackSocUnderwarn_AflThrld  aff_threshold=DEMc_PackSocUnderwarn_AffThrld
      settings: AttributesFormatString=[AFL_INCREMENT=%<afl_inc>]\n[AFL_DECREMENT=%<afl_dec>]\n[AFL_THRESHOLD=%<afl_threshold>]\n[AFF_THRESHOLD=%<aff_threshold>]
  cfault : Outport  OutDataType=fixdt(1, 16)  OutScaling=2^0
  wires:
  diagnostic1/3 -> Terminator2/1
  diagnostic1/4 -> Terminator1/1
  diagnostic1/1 -> Terminator/1
  diagnostic1/2 -> cfault/1
  ifault/1 -> diagnostic1/1

== system DEM_lib/Diagnostic_Event_Management/fault_collect/BPN_Fault_Confirmed/Subsystem24 ==
  ifault : Inport  OutDataType=fixdt(1, 16)  OutScaling=2^0
  Terminator : Terminator
  Terminator1 : Terminator
  Terminator2 : Terminator
  diagnostic1 : Defined_Functionality/diagnostic1  SystemSampleTime=-1  afl_inc=DEMc_PackSocUnderfault_inc  afl_dec=DEMc_PackSocUnderfault_dec  afl_threshold=DEMc_PackSocUnderfault_AflThrld  aff_threshold=DEMc_PackSocUnderfault_AffThrld
      settings: AttributesFormatString=[AFL_INCREMENT=%<afl_inc>]\n[AFL_DECREMENT=%<afl_dec>]\n[AFL_THRESHOLD=%<afl_threshold>]\n[AFF_THRESHOLD=%<aff_threshold>]
  cfault : Outport  OutDataType=fixdt(1, 16)  OutScaling=2^0
  wires:
  ifault/1 -> diagnostic1/1
  diagnostic1/2 -> cfault/1
  diagnostic1/1 -> Terminator/1
  diagnostic1/4 -> Terminator1/1
  diagnostic1/3 -> Terminator2/1

== system DEM_lib/Diagnostic_Event_Management/fault_collect/BPN_Fault_Confirmed/Subsystem25 ==
  ifault : Inport  OutDataType=fixdt(1, 16)  OutScaling=2^0
  Terminator : Terminator
  Terminator1 : Terminator
  Terminator2 : Terminator
  diagnostic1 : Defined_Functionality/diagnostic1  SystemSampleTime=-1  afl_inc=DEMc_PackSocOverwarn_inc  afl_dec=DEMc_PackSocOverwarn_dec  afl_threshold=DEMc_PackSocOverwarn_AflThrld  aff_threshold=DEMc_PackSocOverwarn_AffThrld
      settings: AttributesFormatString=[AFL_INCREMENT=%<afl_inc>]\n[AFL_DECREMENT=%<afl_dec>]\n[AFL_THRESHOLD=%<afl_threshold>]\n[AFF_THRESHOLD=%<aff_threshold>]
  cfault : Outport  OutDataType=fixdt(1, 16)  OutScaling=2^0
  wires:
  diagnostic1/3 -> Terminator2/1
  diagnostic1/4 -> Terminator1/1
  diagnostic1/1 -> Terminator/1
  diagnostic1/2 -> cfault/1
  ifault/1 -> diagnostic1/1

== system DEM_lib/Diagnostic_Event_Management/fault_collect/BPN_Fault_Confirmed/Subsystem26 ==
  ifault : Inport  OutDataType=fixdt(1, 16)  OutScaling=2^0
  Terminator : Terminator
  Terminator1 : Terminator
  Terminator2 : Terminator
  diagnostic1 : Defined_Functionality/diagnostic1  SystemSampleTime=-1  afl_inc=DEMc_PackSocOverfault_inc  afl_dec=DEMc_PackSocOverfault_dec  afl_threshold=DEMc_PackSocOverfault_AflThrld  aff_threshold=DEMc_PackSocOverfault_AffThrld
      settings: AttributesFormatString=[AFL_INCREMENT=%<afl_inc>]\n[AFL_DECREMENT=%<afl_dec>]\n[AFL_THRESHOLD=%<afl_threshold>]\n[AFF_THRESHOLD=%<aff_threshold>]
  cfault : Outport  OutDataType=fixdt(1, 16)  OutScaling=2^0
  wires:
  ifault/1 -> diagnostic1/1
  diagnostic1/2 -> cfault/1
  diagnostic1/1 -> Terminator/1
  diagnostic1/4 -> Terminator1/1
  diagnostic1/3 -> Terminator2/1

== system DEM_lib/Diagnostic_Event_Management/fault_collect/BPN_Fault_Confirmed/Subsystem27 ==
  ifault : Inport  OutDataType=fixdt(1, 16)  OutScaling=2^0
  Terminator : Terminator
  Terminator1 : Terminator
  Terminator2 : Terminator
  diagnostic1 : Defined_Functionality/diagnostic1  SystemSampleTime=-1  afl_inc=DEMc_PulChaPowOverwarn_inc  afl_dec=DEMc_PulChaPowOverwarn_dec  afl_threshold=DEMc_PulChaPowOverwarn_AflThrld  aff_threshold=DEMc_PulChaPowOverwarn_AffThrld
      settings: AttributesFormatString=[AFL_INCREMENT=%<afl_inc>]\n[AFL_DECREMENT=%<afl_dec>]\n[AFL_THRESHOLD=%<afl_threshold>]\n[AFF_THRESHOLD=%<aff_threshold>]
  cfault : Outport  OutDataType=fixdt(1, 16)  OutScaling=2^0
  wires:
  diagnostic1/3 -> Terminator2/1
  diagnostic1/4 -> Terminator1/1
  diagnostic1/1 -> Terminator/1
  diagnostic1/2 -> cfault/1
  ifault/1 -> diagnostic1/1

== system DEM_lib/Diagnostic_Event_Management/fault_collect/BPN_Fault_Confirmed/Subsystem28 ==
  ifault : Inport  OutDataType=fixdt(1, 16)  OutScaling=2^0
  Terminator : Terminator
  Terminator1 : Terminator
  Terminator2 : Terminator
  diagnostic1 : Defined_Functionality/diagnostic1  SystemSampleTime=-1  afl_inc=DEMc_PulChaPowOverfault_inc  afl_dec=DEMc_PulChaPowOverfault_dec  afl_threshold=DEMc_PulChaPowOverfault_AflThrld  aff_threshold=DEMc_PulChaPowOverfault_AffThrld
      settings: AttributesFormatString=[AFL_INCREMENT=%<afl_inc>]\n[AFL_DECREMENT=%<afl_dec>]\n[AFL_THRESHOLD=%<afl_threshold>]\n[AFF_THRESHOLD=%<aff_threshold>]
  cfault : Outport  OutDataType=fixdt(1, 16)  OutScaling=2^0
  wires:
  ifault/1 -> diagnostic1/1
  diagnostic1/2 -> cfault/1
  diagnostic1/1 -> Terminator/1
  diagnostic1/4 -> Terminator1/1
  diagnostic1/3 -> Terminator2/1

== system DEM_lib/Diagnostic_Event_Management/fault_collect/BPN_Fault_Confirmed/Subsystem29 ==
  ifault : Inport  OutDataType=fixdt(1, 16)  OutScaling=2^0
  Terminator : Terminator
  Terminator1 : Terminator
  Terminator2 : Terminator
  diagnostic1 : Defined_Functionality/diagnostic1  SystemSampleTime=-1  afl_inc=DEMc_PulChaPowOverfatal_inc  afl_dec=DEMc_PulChaPowOverfatal_dec  afl_threshold=DEMc_PulChaPowOverfatal_AflThrld  aff_threshold=DEMc_PulChaPowOverfatal_AffThrld
      settings: AttributesFormatString=[AFL_INCREMENT=%<afl_inc>]\n[AFL_DECREMENT=%<afl_dec>]\n[AFL_THRESHOLD=%<afl_threshold>]\n[AFF_THRESHOLD=%<aff_threshold>]
  cfault : Outport  OutDataType=fixdt(1, 16)  OutScaling=2^0
  wires:
  diagnostic1/3 -> Terminator2/1
  diagnostic1/4 -> Terminator1/1
  diagnostic1/1 -> Terminator/1
  diagnostic1/2 -> cfault/1
  ifault/1 -> diagnostic1/1

== system DEM_lib/Diagnostic_Event_Management/fault_collect/BPN_Fault_Confirmed/Subsystem3 ==
  ifault : Inport  OutDataType=fixdt(1, 16)  OutScaling=2^0
  Terminator : Terminator
  Terminator1 : Terminator
  Terminator2 : Terminator
  diagnostic1 : Defined_Functionality/diagnostic1  SystemSampleTime=-1  afl_inc=DEMc_CellVoltOverfault_inc  afl_dec=DEMc_CellVoltOverfault_dec  afl_threshold=DEMc_CellVoltOverfault_AflThrld  aff_threshold=DEMc_CellVoltOverfault_AffThrld
      settings: AttributesFormatString=[AFL_INCREMENT=%<afl_inc>]\n[AFL_DECREMENT=%<afl_dec>]\n[AFL_THRESHOLD=%<afl_threshold>]\n[AFF_THRESHOLD=%<aff_threshold>]
  cfault : Outport  OutDataType=fixdt(1, 16)  OutScaling=2^0
  wires:
  diagnostic1/3 -> Terminator2/1
  diagnostic1/4 -> Terminator1/1
  diagnostic1/1 -> Terminator/1
  diagnostic1/2 -> cfault/1
  ifault/1 -> diagnostic1/1

== system DEM_lib/Diagnostic_Event_Management/fault_collect/BPN_Fault_Confirmed/Subsystem30 ==
  ifault : Inport  OutDataType=fixdt(1, 16)  OutScaling=2^0
  Terminator : Terminator
  Terminator1 : Terminator
  Terminator2 : Terminator
  diagnostic1 : Defined_Functionality/diagnostic1  SystemSampleTime=-1  afl_inc=DEMc_PulDchPowOverwarn_inc  afl_dec=DEMc_PulDchPowOverwarn_dec  afl_threshold=DEMc_PulDchPowOverwarn_AflThrld  aff_threshold=DEMc_PulDchPowOverwarn_AffThrld
      settings: AttributesFormatString=[AFL_INCREMENT=%<afl_inc>]\n[AFL_DECREMENT=%<afl_dec>]\n[AFL_THRESHOLD=%<afl_threshold>]\n[AFF_THRESHOLD=%<aff_threshold>]
  cfault : Outport  OutDataType=fixdt(1, 16)  OutScaling=2^0
  wires:
  ifault/1 -> diagnostic1/1
  diagnostic1/2 -> cfault/1
  diagnostic1/1 -> Terminator/1
  diagnostic1/4 -> Terminator1/1
  diagnostic1/3 -> Terminator2/1

== system DEM_lib/Diagnostic_Event_Management/fault_collect/BPN_Fault_Confirmed/Subsystem31 ==
  ifault : Inport  OutDataType=fixdt(1, 16)  OutScaling=2^0
  Terminator : Terminator
  Terminator1 : Terminator
  Terminator2 : Terminator
  diagnostic1 : Defined_Functionality/diagnostic1  SystemSampleTime=-1  afl_inc=DEMc_PulDchPowOverfault_inc  afl_dec=DEMc_PulDchPowOverfault_dec  afl_threshold=DEMc_PulDchPowOverfault_AflThrld  aff_threshold=DEMc_PulDchPowOverfault_AffThrld
      settings: AttributesFormatString=[AFL_INCREMENT=%<afl_inc>]\n[AFL_DECREMENT=%<afl_dec>]\n[AFL_THRESHOLD=%<afl_threshold>]\n[AFF_THRESHOLD=%<aff_threshold>]
  cfault : Outport  OutDataType=fixdt(1, 16)  OutScaling=2^0
  wires:
  diagnostic1/3 -> Terminator2/1
  diagnostic1/4 -> Terminator1/1
  diagnostic1/1 -> Terminator/1
  diagnostic1/2 -> cfault/1
  ifault/1 -> diagnostic1/1

== system DEM_lib/Diagnostic_Event_Management/fault_collect/BPN_Fault_Confirmed/Subsystem32 ==
  ifault : Inport  OutDataType=fixdt(1, 16)  OutScaling=2^0
  Terminator : Terminator
  Terminator1 : Terminator
  Terminator2 : Terminator
  diagnostic1 : Defined_Functionality/diagnostic1  SystemSampleTime=-1  afl_inc=DEMc_PulDchPowOverfatal_inc  afl_dec=DEMc_PulDchPowOverfatal_dec  afl_threshold=DEMc_PulDchPowOverfatal_AflThrld  aff_threshold=DEMc_PulDchPowOverfatal_AffThrld
      settings: AttributesFormatString=[AFL_INCREMENT=%<afl_inc>]\n[AFL_DECREMENT=%<afl_dec>]\n[AFL_THRESHOLD=%<afl_threshold>]\n[AFF_THRESHOLD=%<aff_threshold>]
  cfault : Outport  OutDataType=fixdt(1, 16)  OutScaling=2^0
  wires:
  ifault/1 -> diagnostic1/1
  diagnostic1/2 -> cfault/1
  diagnostic1/1 -> Terminator/1
  diagnostic1/4 -> Terminator1/1
  diagnostic1/3 -> Terminator2/1

== system DEM_lib/Diagnostic_Event_Management/fault_collect/BPN_Fault_Confirmed/Subsystem33 ==
  ifault : Inport  OutDataType=fixdt(1, 16)  OutScaling=2^0
  Terminator : Terminator
  Terminator1 : Terminator
  Terminator2 : Terminator
  diagnostic1 : Defined_Functionality/diagnostic1  SystemSampleTime=-1  afl_inc=DEMc_PackInnerRfatal_inc  afl_dec=DEMc_PackInnerRfatal_dec  afl_threshold=DEMc_PackInnerRfatal_AflThrld  aff_threshold=DEMc_PackInnerRfatal_AffThrld
      settings: AttributesFormatString=[AFL_INCREMENT=%<afl_inc>]\n[AFL_DECREMENT=%<afl_dec>]\n[AFL_THRESHOLD=%<afl_threshold>]\n[AFF_THRESHOLD=%<aff_threshold>]
  cfault : Outport  OutDataType=fixdt(1, 16)  OutScaling=2^0
  wires:
  diagnostic1/3 -> Terminator2/1
  diagnostic1/4 -> Terminator1/1
  diagnostic1/1 -> Terminator/1
  diagnostic1/2 -> cfault/1
  ifault/1 -> diagnostic1/1

== system DEM_lib/Diagnostic_Event_Management/fault_collect/BPN_Fault_Confirmed/Subsystem34 ==
  ifault : Inport  OutDataType=fixdt(1, 16)  OutScaling=2^0
  Terminator : Terminator
  Terminator1 : Terminator
  Terminator2 : Terminator
  diagnostic1 : Defined_Functionality/diagnostic1  SystemSampleTime=-1  afl_inc=DEMc_PackVoltDropfatal_inc  afl_dec=DEMc_PackVoltDropfatal_dec  afl_threshold=DEMc_PackVoltDropfatal_AflThrld  aff_threshold=DEMc_PackVoltDropfatal_AffThrld
      settings: AttributesFormatString=[AFL_INCREMENT=%<afl_inc>]\n[AFL_DECREMENT=%<afl_dec>]\n[AFL_THRESHOLD=%<afl_threshold>]\n[AFF_THRESHOLD=%<aff_threshold>]
  cfault : Outport  OutDataType=fixdt(1, 16)  OutScaling=2^0
  wires:
  ifault/1 -> diagnostic1/1
  diagnostic1/2 -> cfault/1
  diagnostic1/1 -> Terminator/1
  diagnostic1/4 -> Terminator1/1
  diagnostic1/3 -> Terminator2/1

== system DEM_lib/Diagnostic_Event_Management/fault_collect/BPN_Fault_Confirmed/Subsystem35 ==
  ifault : Inport  OutDataType=fixdt(1, 16)  OutScaling=2^0
  Terminator : Terminator
  Terminator1 : Terminator
  Terminator2 : Terminator
  diagnostic1 : Defined_Functionality/diagnostic1  SystemSampleTime=-1  afl_inc=DEMc_HVPosCtrlRfault_inc  afl_dec=DEMc_HVPosCtrlRfault_dec  afl_threshold=DEMc_HVPosCtrlRfault_AflThrld  aff_threshold=DEMc_HVPosCtrlRfault_AffThrld
      settings: AttributesFormatString=[AFL_INCREMENT=%<afl_inc>]\n[AFL_DECREMENT=%<afl_dec>]\n[AFL_THRESHOLD=%<afl_threshold>]\n[AFF_THRESHOLD=%<aff_threshold>]
  cfault : Outport  OutDataType=fixdt(1, 16)  OutScaling=2^0
  wires:
  diagnostic1/3 -> Terminator2/1
  diagnostic1/4 -> Terminator1/1
  diagnostic1/1 -> Terminator/1
  diagnostic1/2 -> cfault/1
  ifault/1 -> diagnostic1/1

== system DEM_lib/Diagnostic_Event_Management/fault_collect/BPN_Fault_Confirmed/Subsystem36 ==
  ifault : Inport  OutDataType=fixdt(1, 16)  OutScaling=2^0
  Terminator : Terminator
  Terminator1 : Terminator
  Terminator2 : Terminator
  diagnostic1 : Defined_Functionality/diagnostic1  SystemSampleTime=-1  afl_inc=DEMc_HVNegCtrlRfault_inc  afl_dec=DEMc_HVNegCtrlRfault_dec  afl_threshold=DEMc_HVNegCtrlRfault_AflThrld  aff_threshold=DEMc_HVNegCtrlRfault_AffThrld
      settings: AttributesFormatString=[AFL_INCREMENT=%<afl_inc>]\n[AFL_DECREMENT=%<afl_dec>]\n[AFL_THRESHOLD=%<afl_threshold>]\n[AFF_THRESHOLD=%<aff_threshold>]
  cfault : Outport  OutDataType=fixdt(1, 16)  OutScaling=2^0
  wires:
  ifault/1 -> diagnostic1/1
  diagnostic1/2 -> cfault/1
  diagnostic1/1 -> Terminator/1
  diagnostic1/4 -> Terminator1/1
  diagnostic1/3 -> Terminator2/1

== system DEM_lib/Diagnostic_Event_Management/fault_collect/BPN_Fault_Confirmed/Subsystem37 ==
  ifault : Inport  OutDataType=fixdt(1, 16)  OutScaling=2^0
  Terminator : Terminator
  Terminator1 : Terminator
  Terminator2 : Terminator
  diagnostic1 : Defined_Functionality/diagnostic1  SystemSampleTime=-1  afl_inc=DEMc_VoltGetDevifault_inc  afl_dec=DEMc_VoltGetDevifault_dec  afl_threshold=DEMc_VoltGetDevifault_AflThrld  aff_threshold=DEMc_VoltGetDevifault_AffThrld
      settings: AttributesFormatString=[AFL_INCREMENT=%<afl_inc>]\n[AFL_DECREMENT=%<afl_dec>]\n[AFL_THRESHOLD=%<afl_threshold>]\n[AFF_THRESHOLD=%<aff_threshold>]
  cfault : Outport  OutDataType=fixdt(1, 16)  OutScaling=2^0
  wires:
  diagnostic1/3 -> Terminator2/1
  diagnostic1/4 -> Terminator1/1
  diagnostic1/1 -> Terminator/1
  diagnostic1/2 -> cfault/1
  ifault/1 -> diagnostic1/1

== system DEM_lib/Diagnostic_Event_Management/fault_collect/BPN_Fault_Confirmed/Subsystem4 ==
  ifault : Inport  OutDataType=fixdt(1, 16)  OutScaling=2^0
  Terminator : Terminator
  Terminator1 : Terminator
  Terminator2 : Terminator
  diagnostic1 : Defined_Functionality/diagnostic1  SystemSampleTime=-1  afl_inc=DEMc_CellVoltOverfatal_inc  afl_dec=DEMc_CellVoltOverfatal_dec  afl_threshold=DEMc_CellVoltOverfatal_AflThrld  aff_threshold=DEMc_CellVoltOverfatal_AffThrld
      settings: AttributesFormatString=[AFL_INCREMENT=%<afl_inc>]\n[AFL_DECREMENT=%<afl_dec>]\n[AFL_THRESHOLD=%<afl_threshold>]\n[AFF_THRESHOLD=%<aff_threshold>]
  cfault : Outport  OutDataType=fixdt(1, 16)  OutScaling=2^0
  wires:
  ifault/1 -> diagnostic1/1
  diagnostic1/2 -> cfault/1
  diagnostic1/1 -> Terminator/1
  diagnostic1/4 -> Terminator1/1
  diagnostic1/3 -> Terminator2/1

== system DEM_lib/Diagnostic_Event_Management/fault_collect/BPN_Fault_Confirmed/Subsystem5 ==
  ifault : Inport  OutDataType=fixdt(1, 16)  OutScaling=2^0
  Terminator : Terminator
  Terminator1 : Terminator
  Terminator2 : Terminator
  diagnostic1 : Defined_Functionality/diagnostic1  SystemSampleTime=-1  afl_inc=DEMc_CellVoltUnderwarn_inc  afl_dec=DEMc_CellVoltUnderwarn_dec  afl_threshold=DEMc_CellVoltUnderwarn_AflThrld  aff_threshold=DEMc_CellVoltUnderwarn_AffThrld
      settings: AttributesFormatString=[AFL_INCREMENT=%<afl_inc>]\n[AFL_DECREMENT=%<afl_dec>]\n[AFL_THRESHOLD=%<afl_threshold>]\n[AFF_THRESHOLD=%<aff_threshold>]
  cfault : Outport  OutDataType=fixdt(1, 16)  OutScaling=2^0
  wires:
  diagnostic1/3 -> Terminator2/1
  diagnostic1/4 -> Terminator1/1
  diagnostic1/1 -> Terminator/1
  diagnostic1/2 -> cfault/1
  ifault/1 -> diagnostic1/1

== system DEM_lib/Diagnostic_Event_Management/fault_collect/BPN_Fault_Confirmed/Subsystem6 ==
  ifault : Inport  OutDataType=fixdt(1, 16)  OutScaling=2^0
  Terminator : Terminator
  Terminator1 : Terminator
  Terminator2 : Terminator
  diagnostic1 : Defined_Functionality/diagnostic1  SystemSampleTime=-1  afl_inc=DEMc_CellVoltUnderfault_inc  afl_dec=DEMc_CellVoltUnderfault_dec  afl_threshold=DEMc_CellVoltUnderfault_AflThrld  aff_threshold=DEMc_CellVoltUnderfault_AffThrld
      settings: AttributesFormatString=[AFL_INCREMENT=%<afl_inc>]\n[AFL_DECREMENT=%<afl_dec>]\n[AFL_THRESHOLD=%<afl_threshold>]\n[AFF_THRESHOLD=%<aff_threshold>]
  cfault : Outport  OutDataType=fixdt(1, 16)  OutScaling=2^0
  wires:
  ifault/1 -> diagnostic1/1
  diagnostic1/2 -> cfault/1
  diagnostic1/1 -> Terminator/1
  diagnostic1/4 -> Terminator1/1
  diagnostic1/3 -> Terminator2/1

== system DEM_lib/Diagnostic_Event_Management/fault_collect/BPN_Fault_Confirmed/Subsystem7 ==
  ifault : Inport  OutDataType=fixdt(1, 16)  OutScaling=2^0
  Terminator : Terminator
  Terminator1 : Terminator
  Terminator2 : Terminator
  diagnostic1 : Defined_Functionality/diagnostic1  SystemSampleTime=-1  afl_inc=DEMc_CellVoltUnderfatal_inc  afl_dec=DEMc_CellVoltUnderfatal_dec  afl_threshold=DEMc_CellVoltUnderfatal_AflThrld  aff_threshold=DEMc_CellVoltUnderfatal_AffThrld
      settings: AttributesFormatString=[AFL_INCREMENT=%<afl_inc>]\n[AFL_DECREMENT=%<afl_dec>]\n[AFL_THRESHOLD=%<afl_threshold>]\n[AFF_THRESHOLD=%<aff_threshold>]
  cfault : Outport  OutDataType=fixdt(1, 16)  OutScaling=2^0
  wires:
  diagnostic1/3 -> Terminator2/1
  diagnostic1/4 -> Terminator1/1
  diagnostic1/1 -> Terminator/1
  diagnostic1/2 -> cfault/1
  ifault/1 -> diagnostic1/1

== system DEM_lib/Diagnostic_Event_Management/fault_collect/BPN_Fault_Confirmed/Subsystem8 ==
  ifault : Inport  OutDataType=fixdt(1, 16)  OutScaling=2^0
  Terminator : Terminator
  Terminator1 : Terminator
  Terminator2 : Terminator
  diagnostic1 : Defined_Functionality/diagnostic1  SystemSampleTime=-1  afl_inc=DEMc_CellVoltDifOverwarn_inc  afl_dec=DEMc_CellVoltDifOverwarn_dec  afl_threshold=DEMc_CellVoltDifOverwarn_AflThrld  aff_threshold=DEMc_CellVoltDifOverwarn_AffThrld
      settings: AttributesFormatString=[AFL_INCREMENT=%<afl_inc>]\n[AFL_DECREMENT=%<afl_dec>]\n[AFL_THRESHOLD=%<afl_threshold>]\n[AFF_THRESHOLD=%<aff_threshold>]
  cfault : Outport  OutDataType=fixdt(1, 16)  OutScaling=2^0
  wires:
  ifault/1 -> diagnostic1/1
  diagnostic1/2 -> cfault/1
  diagnostic1/1 -> Terminator/1
  diagnostic1/4 -> Terminator1/1
  diagnostic1/3 -> Terminator2/1

== system DEM_lib/Diagnostic_Event_Management/fault_collect/BPN_Fault_Confirmed/Subsystem9 ==
  ifault : Inport  OutDataType=fixdt(1, 16)  OutScaling=2^0
  Terminator : Terminator
  Terminator1 : Terminator
  Terminator2 : Terminator
  diagnostic1 : Defined_Functionality/diagnostic1  SystemSampleTime=-1  afl_inc=DEMc_CellVoltDifOverfault_inc  afl_dec=DEMc_CellVoltDifOverfault_dec  afl_threshold=DEMc_CellVoltDifOverfault_AflThrld  aff_threshold=DEMc_CellVoltDifOverfault_AffThrld
      settings: AttributesFormatString=[AFL_INCREMENT=%<afl_inc>]\n[AFL_DECREMENT=%<afl_dec>]\n[AFL_THRESHOLD=%<afl_threshold>]\n[AFF_THRESHOLD=%<aff_threshold>]
  cfault : Outport  OutDataType=fixdt(1, 16)  OutScaling=2^0
  wires:
  diagnostic1/3 -> Terminator2/1
  diagnostic1/4 -> Terminator1/1
  diagnostic1/1 -> Terminator/1
  diagnostic1/2 -> cfault/1
  ifault/1 -> diagnostic1/1

== system DEM_lib/Diagnostic_Event_Management/fault_collect/BSC_Fault_Confirmed/Subsystem2 ==
  ifault : Inport  OutDataType=fixdt(1, 16)  OutScaling=2^0
  Terminator : Terminator
  Terminator1 : Terminator
  Terminator2 : Terminator
  diagnostic1 : Defined_Functionality/diagnostic1  SystemSampleTime=-1  afl_inc=1  afl_dec=2  afl_threshold=10  aff_threshold=255
      settings: AttributesFormatString=[AFL_INCREMENT=%<afl_inc>]\n[AFL_DECREMENT=%<afl_dec>]\n[AFL_THRESHOLD=%<afl_threshold>]\n[AFF_THRESHOLD=%<aff_threshold>]
  cfault : Outport  OutDataType=fixdt(1, 16)  OutScaling=2^0
  wires:
  diagnostic1/3 -> Terminator2/1
  diagnostic1/4 -> Terminator1/1
  diagnostic1/1 -> Terminator/1
  diagnostic1/2 -> cfault/1
  ifault/1 -> diagnostic1/1
